simulink model "demo_simplemodel"
settings: Solver=ode1  SolverMode=SingleTasking  StartTime=0.0  StopTime=inf  FixedStep=0.001  RelTol=1e-3  AbsTol=1e-6
PostLoadFcn:
  | , if any(exist('dsrtsu_mdlpostloadfcn', 'file') == [2, 3, 6]), try dsrtsu_mdlpostloadfcn('Execute', bdroot); catch fprintf('Error in PostLoadFcn (dsrtsu_mdlpostloadfcn) for model "%s":\n %s\n', bdroot, lasterr); end, end,
undefined symbols (not defined in the file or in its folder): rticanmm_blockfcn, rticanmm_initfcn
libraries: rtimmsu_dsrtlib x2
settings Model: RTICANMMDATA=struct('GeneralSetupData',struct('modelroot','E:\projects\dSPACE-RLS-Variants\current\RTICANMM\Components\Demos\RTICANMM\simplemodel','generalsettings',struct('filesettings',struct('destfolder',struct('Name','RTICANMM_FILES','Check',1),'buildfolder',struct('Name','.','Check',1),'AbsDestfolder',struct('Name','E:\projects\dSPACE-RLS-Variants\current\RTICANMM\Components\Demos\RTICANMM\simplemodel\RTICANMM_FILES'),'AbsBuildfolder',struct('Name','E:\projects\dSPACE-RLS-Variants\current\RTICANMM\Components\Demos\RTICANMM\simplemodel'))),'options',struct('addpaths',1,'rmpaths',1,'addtrcexclusion',1,'cannavigator',struct('checkmonitoring',0,'serviceno','31','hostservicedefheader',struct('name','RTICANMMHostService_demo_simplemodel.h','path','D:\Sandboxes\dSPACE-Releases\6.7\RTICANMM\Components\Demos\RTICANMM\simplemodel\RTICANMM_FILES\RTICANMMHostService_demo_simplemodel.h'),'checkinternmonitoring',1),'show_usrtrc',0,'use_usrtrc',0,'addpath2usrmk',1),'advanced',struct('options',[1 1 1 1 1 1 1 1 1 1 1 1 1 1 1 1 1 1 1 1 1 1 1 1 1 1 1 1 1 1 1 1 1 1 1 1 1 1 1 1 1 1 1 1 1 1 1 1 1 1 1 1 1 1 1 1 1 1 1 1 1 1 1 1 1 1 1 1 1 1 1 1 1 1 1 1 1 1 1 1 1 1 1 1 1 1 1 1 1 1 1 1 1 1 1 1 1 1 1 1]),'MPSetup',{{}},'RTI',struct('Type','RTI1005','Ver','7.1','Date','02-Nov-2013'),'version','3.0.735627.5512384259','modelname','demo_simplemodel','userdata',struct('CANMMName',{{'CAN'}},'HostServiceChannelID',{{[],'CAN_Controller_1'}}),'block',['demo_simplemodel/RTICANMM' char(10) 'GeneralSetup'],'GetDataFromRTICANMM',0,'allgeneratedfiles',{{'D:\Sandboxes\dSPACE-Releases\6.7\RTICANMM\Components\Demos\RTICANMM\simplemodel\RTICANMM_FILES\RTICANMMHostService_demo_simplemodel.h','D:\projects\dSPACE-RLS-Variants\6.5\RTICANMM\Components\Demos\RTICANMM\simplemodel\RTICANMM_FILES\RTICANMMHostService_demo_simplemodel.h'}},'MMType','RTICANMM'),'BuildData',struct('GeneralSetupData',struct('modelroot','d:\tmp\Demos\simplemodel','generalsettings',struct('filesettings',struct('destfolder',struct('Name','RTICANMM_FILES','Check',1),'buildfolder',struct('Name','.','Check',1),'AbsDestfolder',struct('Name','d:\tmp\Demos\simplemodel\RTICANMM_FILES'),'AbsBuildfolder',struct('Name','d:\tmp\Demos\simplemodel'))),'options',struct('addpaths',1,'rmpaths',1,'addtrcexclusion',1,'cannavigator',struct('checkmonitoring',0,'checkinternmonitoring',1,'serviceno','31','hostservicedefheader',struct('name','RTICANMMHostService_demo_simplemodel.h','path','d:\tmp\Demos\simplemodel\RTICANMM_FILES\RTICANMMHostService_demo_simplemodel.h')),'use_usrtrc',0,'addpath2usrmk',1),'advanced',struct('options',[1 1 1 1 1 1 1 1 1 1 1 1 1 1 1 1 1 1 1 1 1 1 1 1 1 1 1 1 1 1 1 1 1 1 1 1 1 1 1 1 1 1 1 1 1 1 1 1 1 1 1 1 1 1 1 1 1 1 1 1 1 1 1 1 1 1 1 1 1 1 1 1 1 1 1 1 1 1 1 1 1 1 1 1 1 1 1 1 1 1 1 1 1 1 1 1 1 1 1 1]),'MPSetup',{{}},'RTI',struct('Type','RTI1005','Ver','6.1f8','Date','19-Jun-2008'),'version','2.4b1.733561.482','modelname','demo_simplemodel','userdata',struct('CANMMName',{{'CAN'}}),'block',['demo_simplemodel/RTICANMM' char(10) 'GeneralSetup'],'GetDataFromRTICANMM',0),'ModelBuildIsUpToDate',0,'ModelCurrentSDFFile','D:\projects\dSPACE-RLS-Variants\current\RTICANMM\Components\Demos\RTICANMM\simplemodel\demo_simplemodel.sdf'))  RTILINMMDATA=struct('GeneralSetupData',[])  DSRTSU_INTERNAL_RTI_VER=430  DSRTSU_INTERNAL_RTI_TYPE=rti1005  DSRTSU_INTERNAL_RTIFLEXRAYCONFIG=60  DSRTSU_INTERNAL_RTIFPGA=30  ExtModeTrigMode=oneshot  ExtModeArmWhenConnect=off  BufferReuse=off  Creator=dSPACE GmbH  LastModifiedBy=dSPACE GmbH
settings DataIOCC: SaveFormat=Array  SignalLoggingSaveFormat=ModelDataLogs  ReturnWorkspaceOutputs=off  SignalLoggingName=sigsOut
settings OptimizationCC: BlockReduction=off  ConditionallyExecuteInputs=off  OptimizeBlockIOStorage=off  BufferReuse=off  ExpressionFolding=off  ExpressionDepthLimit=2147483647  FoldNonRolledExpr=off  LocalBlockOutputs=off  InitFltsAndDblsToZero=on  LifeSpan=inf  SimCompilerOptimization=Off
settings DebuggingCC: SaveWithParameterizedLinksMsg=none  UnderspecifiedInitializationDetection=Classic  MergeDetectMultiDrivingBlocksExec=none  SignalResolutionControl=TryResolveAllWithWarning  InheritedTsInSrcMsg=none  MultiTaskDSMMsg=warning  MultiTaskCondExecSysMsg=none  FcnCallInpInsideContextMsg=Use local settings  FrameProcessingCompatibilityMsg=warning  StateNameClashWarn=warning  SFUnexpectedBacktrackingDiag=warning  SFNoUnconditionalDefaultTransitionDiag=warning
settings HardwareCC: ProdBitPerPointer=32  ProdLargestAtomicFloat=None  ProdEndianess=BigEndian  ProdWordSize=32  ProdHWDeviceType=Generic->Custom  TargetIntDivRoundTo=Zero  TargetEndianess=BigEndian  TargetHWDeviceType=Generic->Custom
settings ModelReferenceCC: PropagateSignalLabelsOutOfModel=off
settings SFSimCC: SimUseLocalCustomCode=off
settings RTWCC: SystemTargetFile=rti1005.tlc  MakeCommand=make_rti  TemplateMakefile=rti1005.tmf  RTWVerbose=off  RetainRTWFile=on  ProcessScript=rti1005_make_rtw_hook  RTWUseLocalCustomCode=off  RTWCompilerOptimization=Off
settings CodeAppCC: IncHierarchyInIds=on  CustomSymbolStrType=$N$R$M  CustomSymbolStrField=$H$N$M  CustomSymbolStrFcn=$R$H$N$M$F
settings STFCustomTargetCC: TargetFcnLib=ansi_tfl_tmw.mat  CodeReplacementLibrary=ANSI_C  ParMdlRefBuildCompliant=on  GeneratePreprocessorConditionals=Disable all  SystemTargetFile=rti1005.tlc
settings GRTTargetCC: TargetFcnLib=ansi_tfl_tmw.mat  CodeReplacementLibrary=ANSI_C  CompOptLevelCompliant=off  ConcurrentExecutionCompliant=off  GeneratePreprocessorConditionals=Disable all  CombineOutputUpdateFcns=off  MatFileLogging=off  CPPClassGenCompliant=off  GRTInterface=on  ExtMode=on  ExtModeMexFile=noextcomm

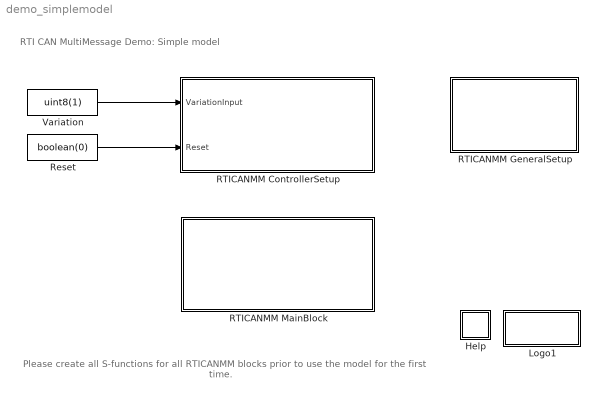
== system demo_simplemodel ==
  note: RTI CAN MultiMessage Demo: Simple model
  note: Please create all S-functions for all RTICANMM blocks prior to use the model for the first time.
  Help : Subsystem
      mask Display: disp('?');
  Logo1 : Subsystem  mask(dSPACE){EmptyParameter=[]}
      mask prompts: EmptyParameter "Mask Parameter 1:"
      settings: OpenFcn=;
      mask Display: image(imread('rti_mdl_dslogo.tif'));
  RTICANMM ControllerSetup : Subsystem  InitFcn=rticanmm_blockfcn('InitFcn', 'CANnedySetup', gcb)  ClipboardFcn=rticanmm_blockfcn('ClipboardFcn', 'CANnedySetup', gcb)  mask(RTICANMM){DSProperties=struct('RTI',struct('Version',uint32(1),'BlockType',struct('isSLSource',uint8(1),'isSLSink',uint8(1),'isHWSource',uint8(0),'isHWSink',uint8(0),'isSetup',uint8(0),'isInline',uint8(1),'isNonInline',uint8(0),'isInterrupt',uint8(0),'isChannelwise',uint8(0)),'IOBoardType','RTICANMM','UnitType','RTICANMM','Identifier','BUSSETUP','DialogType','SL','BlockSet','RTICANMM','SlaveProcessor','CAN')), CANMMProperties=struct('cannedy',struct('data',struct('options',struct('controllername','CAN_Controller_1','controllernameautomatic',[],'loglevel','0','checkrealtime',0,'checkchangebaudrate',0,'sampletime','1','CANControllerStatus',0,'NumberofStuffErr',0,'NumberofFormErr',0,'NumberofAckErr',0,'NumberofBit0Err',0,'NumberofsuccrecRX',0,'Numberofsuccsent',0,'NumberofBit1Err',0,'NumberofCRCErr',0,'NumberoflostRX',0,'Busoff',0,'Busload',0,'OperationPending',0,'TxRetryCount',3,'addtrcexclusion',logical(1),'cannavigator',struct('checkmonitoring',0,'checkinternmonitoring',0),'show_usrtrc',0,'use_usrtrc',0),'modelroot','d:\\temp\\RTICANMM\\simplemodel','generalsettings',struct('setupdata',struct('board','DS4302','boardno',1,'channelno',1,'Type','STD','transceiver','ISO11898-2','busconfig','0x0','feedthrough','false','resistance',struct('r120',1,'roff',0,'r16',1,'r10',0),'baudrate','500','Frequency',[24 36],'samplemode',1,'commChannelTJA1041',6,'config',struct('standard',1,'advanced',0,'register',struct('btr0','0x40','btr1','0x1C','sp','87','sjw','1','tseg1','12','tseg2','1','brp','0','smpl','0','btr0_36','0x40','btr1_36','0x1C','sp_36','87','sjw_36','1','tseg1_36','12','tseg2_36','1','brp_36','0','smpl_36','0','btr0_64','0x40','btr1_64','0x1C','sp_64','87','sjw_64','1','tseg1_64','12','tseg2_64','1','brp_64','0','smpl_64','0')),'channelcfg',struct('INTENDISABLE','CAN_INT_DISABLE','intenable',0),'SETUPID','RTICANMM_CAN_Controller_1_ID','CONTROLLER_ID','CANMM_CTL_SETUP_CAN_Controller_1','mainblock_includefile','RTICANMM_SETUP_CAN_Controller_1','termination','TERMINATION_ON'),'filesettings',struct('destfolder',struct('Name','RTICANMM_FILES','Check',1),'buildfolder',struct('Name','.','Check',1))),'advanced',struct('options',[1 1 1 1 1 1 1 1 1 1 1 1 1 1 1 1 1 1 1 1 1 1 1 1 1 1 1 1 1 1 1 1 1 1 1 1 1 1 1 1 1 1 1 1 1 1 1 1 1 1 1 1 1 1 1 1 1 1 1 1 1 1 1 1 1 1 1 1 1 1 1 1 1 1 1 1 1 1 1 1 1 1 1 1 1 1 1 1 1 1 1 1 1 1 1 1 1 1 1 1]),'partialnetdata',struct('switchedon',0,'format','STD','idmask',['XXXXX XXXXXXXX XXXXXXXX XXXXXXXX'],'idcode','0','idfilter','0','datamaskused',0,'datalength','0','datamask','0x0000000000000000','partialnetworkenable',0)),'blk',['demo_simplemodel/RTICANMM' char(10) 'ControllerSetup'],'allgeneratedfiles',{{'E:\\projects\\dSPACE-RLS-Variants\\current\\RTICANMM\\Components\\Demos\\RTICANMM\\simplemodel\\RTICANMM_FILES\\RTICANMM_SETUP_CAN_Controller_1.c','E:\\projects\\dSPACE-RLS-Variants\\current\\RTICANMM\\Components\\Demos\\RTICANMM\\simplemodel\\RTICANMM_FILES\\RTICANMM_SETUP_CAN_Controller_1.h','e:\\projects\\dspace-rls-variants\\current\\rticanmm\\components\\demos\\rticanmm\\simplemodel\\rticanmm_files\\rticanmm_setup_can_controller_1.mexw32'}},'ismp',logical(0),'BlockDataVersion','0.6.0','recreate',0),'CANnedynew',0,'CANnedySettings','CAN_Controller_1','GeneratedFiles',{{'E:\\projects\\dSPACE-RLS-Variants\\current\\RTICANMM\\Components\\Demos\\RTICANMM\\simplemodel\\RTICANMM_FILES\\RTICANMM_SETUP_CAN_Controller_1.c','E:\\projects\\dSPACE-RLS-Variants\\current\\RTICANMM\\Components\\Demos\\RTICANMM\\simplemodel\\RTICANMM_FILES\\RTICANMM_SETUP_CAN_Controller_1.h','e:\\projects\\dspace-rls-variants\\current\\rticanmm\\components\\demos\\rticanmm\\simplemodel\\rticanmm_files\\rticanmm_setup_can_controller_1.mexw32'}},'SFCN','RTICANMM_SETUP_CAN_Controller_1.c','HostService',struct('Tags',struct('DATA','RTICANMM_MonitorData','Enable','CANMMMonitor_CAN_Controller_1','TimeStamp','MonitoringTimeStamp_CAN_Controller_1'),'DATA',struct('Length',4),'Info',struct('Desc',{'ID','Service','Data1','Data2'}),'Names',struct('Enable','Monitoring_Enable','TimeStamp','Monitoring_TimeStamp'),'ChannelID',2)), CANMMType=CANnedySetup, CANMMFolder=E:\\projects\\dSPACE-RLS-Variants\\current\\RTICANMM\\Components\\Demos\\RTICANMM\\simplemodel, CANMMDestFolder=RTICANMM_FILES, CANMMSettings=CAN_Controller_1, CANMMSFcn=RTICANMM_SETUP_CAN_Controller_1, CANMMBoard=DS4302, CANMMBoardNum=1, CANMMChannel=1}
      settings: AttributesFormatString=%<CANMMSettings>: %<CANMMBoard>_B%<CANMMBoardNum>_C%<CANMMChannel>  CopyFcn=rticanmm_blockfcn('CopyFcn', 'CANnedySetup', gcb)  DeleteFcn=rticanmm_blockfcn('DeleteFcn', 'CANnedySetup', gcb)  ModelCloseFcn=rticanmm_blockfcn('ModelCloseFcn', 'CANnedySetup', gcb)  NameChangeFcn=rticanmm_blockfcn('NameChangeFcn', 'CANnedySetup', gcb)  OpenFcn=try, rticanmm_setup_gui('create',gcb); ; catch,errordlg({lasterr, '','Please check your RTI installation.'},['Error: ' upper(bdroot)], 'replace'); end  MoveFcn=rticanmm_blockfcn('MoveFcn', 'CANnedySetup', gcb)
      mask Help: eval('rticanmm_quickstart(''create'', gcb);', 'disp(lasterr);')
      mask Display:
      | disp('RTI CAN\nMultiMessage\nControllerSetup')
      | 
      | port_label('input', 1 , 'Variation')
      | port_label('input', 2 , 'Reset')
  RTICANMM GeneralSetup : Subsystem  InitFcn=rticanmm_initfcn(gcb, 'CANnedySettings')  ClipboardFcn=rticanmm_blockfcn('ClipboardFcn', 'CANnedySettings', gcb)  mask(RTICANMM){DSProperties=struct('RTI',struct('Version',uint32(1),'BlockType',struct('isSLSource',uint8(1),'isSLSink',uint8(1),'isHWSource',uint8(0),'isHWSink',uint8(0),'isSetup',uint8(0),'isInline',uint8(1),'isNonInline',uint8(0),'isInterrupt',uint8(0),'isChannelwise',uint8(0)),'IOBoardType','RTICANMM','UnitType','RTICANMM','Identifier','GENERALSETUP','DialogType','SL','BlockSet','RTICANMM','SlaveProcessor','CAN')), CANMMDestFolder=RTICANMM_FILES, CANMMBuildDir=., CANMMAddPaths=on, CANMMAddpathUserMake=on, CANMMRemovePathOnclose=on, CANMMType=CANnedySettings, CANMMProperties=struct('modelroot','E:\\projects\\dSPACE-RLS-Variants\\current\\RTICANMM\\Components\\Demos\\RTICANMM\\simplemodel','generalsettings',struct('filesettings',struct('destfolder',struct('Name','RTICANMM_FILES','Check',1),'buildfolder',struct('Name','.','Check',1),'AbsDestfolder',struct('Name','E:\\projects\\dSPACE-RLS-Variants\\current\\RTICANMM\\Components\\Demos\\RTICANMM\\simplemodel\\RTICANMM_FILES'),'AbsBuildfolder',struct('Name','E:\\projects\\dSPACE-RLS-Variants\\current\\RTICANMM\\Components\\Demos\\RTICANMM\\simplemodel'))),'options',struct('addpaths',1,'rmpaths',1,'addtrcexclusion',1,'cannavigator',struct('checkmonitoring',0,'serviceno','31','hostservicedefheader',struct('name','RTICANMMHostService_demo_simplemodel.h','path','D:\\Sandboxes\\dSPACE-Releases\\6.7\\RTICANMM\\Components\\Demos\\RTICANMM\\simplemodel\\RTICANMM_FILES\\RTICANMMHostService_demo_simplemodel.h'),'checkinternmonitoring',1),'show_usrtrc',0,'use_usrtrc',0,'addpath2usrmk',1),'advanced',struct('options',[1 1 1 1 1 1 1 1 1 1 1 1 1 1 1 1 1 1 1 1 1 1 1 1 1 1 1 1 1 1 1 1 1 1 1 1 1 1 1 1 1 1 1 1 1 1 1 1 1 1 1 1 1 1 1 1 1 1 1 1 1 1 1 1 1 1 1 1 1 1 1 1 1 1 1 1 1 1 1 1 1 1 1 1 1 1 1 1 1 1 1 1 1 1 1 1 1 1 1 1]),'MPSetup',{{}},'RTI',struct('Type','RTI1005','Ver','7.1','Date','02-Nov-2013'),'version','3.0.735627.5512384259','modelname','demo_simplemodel','userdata',struct('CANMMName',{{'CAN'}},'HostServiceChannelID',{{[],'CAN_Controller_1'}}),'block',['demo_simplemodel/RTICANMM' char(10) 'GeneralSetup'],'GetDataFromRTICANMM',0,'allgeneratedfiles',{{'D:\\Sandboxes\\dSPACE-Releases\\6.7\\RTICANMM\\Components\\Demos\\RTICANMM\\simplemodel\\RTICANMM_FILES\\RTICANMMHostService_demo_simplemodel.h','D:\\projects\\dSPACE-RLS-Variants\\6.5\\RTICANMM\\Components\\Demos\\RTICANMM\\simplemodel\\RTICANMM_FILES\\RTICANMMHostService_demo_simplemodel.h'}},'MMType','RTICANMM')}
      mask prompts: CANMMDestFolder "Destination Folder for generated Files:"; CANMMBuildDir "Build Directory (*_usr.mk, *_usr.trc)"; CANMMAddPaths "Add Paths automatically"; CANMMAddpathUserMake "Add Paths to UserMake-File"; CANMMRemovePathOnclose "Remove added Path on ModelClose"
      mask init:
      | rticanmm_initfcn(gcb,'CANnedyGeneralSettings')
      settings: CopyFcn=rticanmm_blockfcn('CopyFcn', 'CANnedySettings', gcb)  DeleteFcn=rticanmm_blockfcn('DeleteFcn', 'CANnedySettings', gcb)  ModelCloseFcn=rticanmm_blockfcn('CloseFcn', 'CANnedyGeneralSettings', gcb)  NameChangeFcn=rticanmm_blockfcn('NameChangeFcn', 'CANnedySettings', gcb)  OpenFcn=try, rticanmm_gs_gui('create',gcb), ; catch,errordlg({lasterr, '','Please check your RTI installation.'},['Error: ' upper(bdroot)], 'replace'); end  MoveFcn=rticanmm_blockfcn('MoveFcn', 'CANnedySettings', gcb)
      mask Help: eval('rticanmm_quickstart(''create'', gcb);', 'disp(lasterr);')
      mask Display: disp(sprintf(['RTI CAN\nMultiMessage\nGeneralSetup']))
  RTICANMM MainBlock : Subsystem  InitFcn=rticanmm_blockfcn('InitFcn', 'CANnedy', gcb)  ClipboardFcn=rticanmm_blockfcn('ClipboardFcn', 'CANnedy', gcb)  mask(RTICANMM){DSProperties=struct('RTI',struct('Version',uint32(1),'BlockType',struct('isSLSource',uint8(1),'isSLSink',uint8(1),'isHWSource',uint8(0),'isHWSink',uint8(0),'isSetup',uint8(0),'isInline',uint8(1),'isNonInline',uint8(0),'isInterrupt',uint8(0),'isChannelwise',uint8(0)),'IOBoardType','RTICANMM','UnitType','RTICANMM','Identifier','Mainblock','DialogType','SL','BlockSet','RTICANMM','SlaveProcessor','CAN')), CANMMProperties=struct('RTICANMMVersion','3.0','RTICANMMVersionIntern','3.0.735627.5512384259','RTICANMMDate','02-May-2014','Settings','RTICANMM_MAIN_CAN','UserTracePath','','ModelPath','E:\\projects\\dSPACE-RLS-Variants\\current\\RTICANMM\\Components\\Demos\\RTICANMM\\simplemodel','filesettings',struct('FileName','RTICANMM_DEMO_DBC.DBC','IsRelative',1,'ClusterId',1,'ClusterList',{{'default'}},'destfolder',struct('Name','RTICANMM_FILES','Check',1),'buildfolder',struct('Name','.','Check',1),'onlyfreerawcapture',0,'overlapping2variant',0),'onlyfreerawcapture',0,'Board','DS4302','BoardNum','1','ChannelNum','1','Variation','1','SetupId','CAN_Controller_1','MARK',['8E4F1C302B791474ADA830CE4B10A2';'10AE92B0A04702328E2FF4C03423CB';'41FF555D4D357435AA3D32256C7A7E';'213C370CD9596A2BAB0FF3FD076AF2';'AECECA6456FE9F581A20B280178641'],'date','03-Feb-2014','clock',['03.02.2014 14:47:55'],'recreate',0,'RTIVER','RTI1005','j1939',0,'TRC',struct('include',1),'rtsupport',struct('XMLFile','E:\\projects\\dSPACE-RLS-Variants\\current\\RTICANMM\\Components\\Demos\\RTICANMM\\simplemodel\\RTICANMM_FILES\\RTICANMM_MAIN_CAN.xml','DBCXML',struct('Path','E:\\projects\\dSPACE-RLS-Variants\\current\\RTICANMM\\Components\\Demos\\RTICANMM\\simplemodel\\RTICANMM_FILES\\RTICANMM_MAIN_CAN_dbc.xml','support',1,'Name','RTICANMM_DEMO_DBC.DBC','Date',['19-Jul-2011 12:20:58'],'Type','mixed','DBCSupport','ON'))), CANMMType=CANnedy, CANMMUserTraceMerged=off, CANMMUserTracePath=, CANMMChannelNum=1, CANMMBoardNum=1, CANMMDestFolder=RTICANMM_FILES, CANMMFolder=., CANMMSetupId=CAN_Controller_1, CANMMsave2mat=['8E4F1C302B791474ADA830CE4B10A2';'10AE92B0A04702328E2FF4C03423CB';'41FF555D4D357435AA3D32256C7A7E';'213C370CD9596A2BAB0FF3FD076AF2';'AECECA6456FE9F581A20B280178641'], CANMMName=CAN, CANMMSettings=RTICANMM_MAIN_CAN, CANMMIntermediateTag=RTICANMM_MAIN_CAN_intermediate, CANMMsfcnname=RTICANMM_MAIN_CAN}
      mask init:
      | rticanmm_initfcn(gcb, CANMMType, CANMMsfcnname)
      settings: AttributesFormatString=CAN_Controller_1[CAN]: DS4302_B1_C1_V1  CopyFcn=rticanmm_blockfcn('CopyFcn', 'CANnedy', gcb)  DeleteFcn=rticanmm_blockfcn('DeleteFcn', 'CANnedy', gcb)  ModelCloseFcn=rticanmm_blockfcn('ModelCloseFcn', 'CANnedy', gcb)  NameChangeFcn=rticanmm_blockfcn('NameChangeFcn', 'CANnedy', gcb)  OpenFcn=try, rticanmm_main_gui('create',gcb); ; catch,errordlg({lasterr, '','Please check your RTI installation.'},['Error: ' upper(bdroot)], 'replace'); end  MoveFcn=rticanmm_blockfcn('MoveFcn', 'CANnedy', gcb)
      mask Help: eval('rticanmm_quickstart(''create'', gcb);', 'disp(lasterr);')
      mask Display: disp(sprintf('RTI CAN\nMultiMessage\nMainSetup'))
  Reset : Constant  Value=boolean(0)
  Variation : Constant  Value=uint8(1)
  wires:
  Variation/1 -> RTICANMM ControllerSetup/1(VariationInput)
  Reset/1 -> RTICANMM ControllerSetup/2(Reset)

== system demo_simplemodel/Help ==
  note: The block named 'General Setup'  defines the folder 'RTICANMM_FILES' as destination
      | folder for all files created by RTICANMM.
  note: The block named 'MainBlock' has been configured by the DBC file 'rticanmm_demo_dbc.dbc'.
  note: This demo model illustrates the usage of the RTI CAN Mulit Message Blockset.
      | The Controller Setup blocks configure the CAN controller for a baudrate of 500 kbit/s.

== system demo_simplemodel/Logo1 ==
  note: $Workfile: demo_rticanmm_simplemodel.mdl $
  note: $Date: 2013/07/08 14:25:20MESZ $
  note: $Revision: 1.33 $

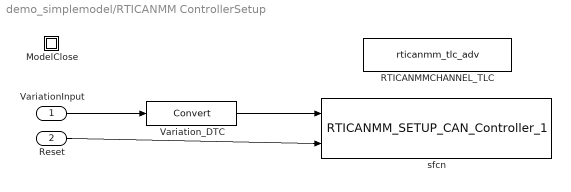
== system demo_simplemodel/RTICANMM ControllerSetup ==
  VariationInput : Inport
  Reset : Inport  Port=2
  ModelClose : Subsystem
      mask Type: RTICANMMModelClose
  RTICANMMCHANNEL_TLC : S-Function  FunctionName=rticanmm_tlc_adv  Parameters=4302,1,1,0,500,'unused'  EnableBusSupport=off
      mask Type: RTICANMMCHANNEL_TLC
  Variation_DTC : DataTypeConversion  SaturateOnIntegerOverflow=on  RndMeth=Zero
  sfcn : S-Function  InitFcn=rticanmm_initfcn(gcb, 'SFCNs')  FunctionName=RTICANMM_SETUP_CAN_Controller_1  EnableBusSupport=off
      mask init:
      | rticanmm_initfcn(gcb, 'SFCNs')
  wires:
  Reset/1 -> sfcn/2
  VariationInput/1 -> Variation_DTC/1
  Variation_DTC/1 -> sfcn/1

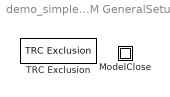
== system demo_simplemodel/RTICANMM GeneralSetup ==
  ModelClose : Subsystem
      mask Type: RTICANMMModelClose
  TRC Exclusion : rtimmsu_dsrtlib/TRC Exclusion

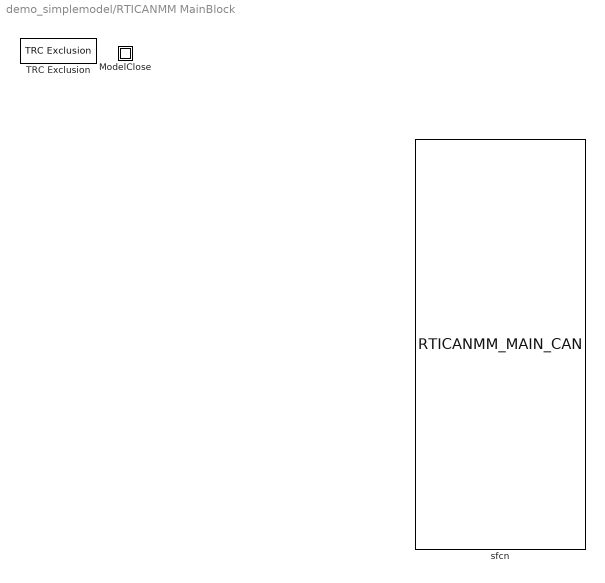
== system demo_simplemodel/RTICANMM MainBlock ==
  ModelClose : Subsystem
      mask Type: RTICANMMModelClose
  TRC Exclusion : rtimmsu_dsrtlib/TRC Exclusion
  sfcn : S-Function  InitFcn=rticanmm_initfcn(gcb, 'SFCNs')  FunctionName=RTICANMM_MAIN_CAN  EnableBusSupport=off
      mask init:
      | rticanmm_initfcn(gcb, 'SFCNs')

== system demo_simplemodel/RTICANMM ControllerSetup/ModelClose ==

== system demo_simplemodel/RTICANMM GeneralSetup/ModelClose ==

== system demo_simplemodel/RTICANMM MainBlock/ModelClose ==
